simulink model "Type2_b"  (R2019a)
settings: Solver=VariableStepAuto  StartTime=0.0  StopTime=10.0  RelTol=1e-3
libraries: simulink x2
settings Model: Creator=admin  LastModifiedBy=admin

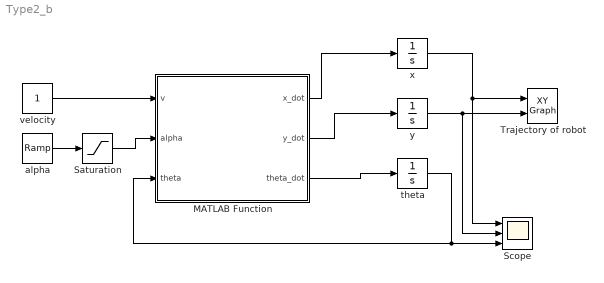
== system Type2_b ==
  MATLAB Function : MATLAB Function  TreatAsAtomicUnit=on
  Saturation : Saturate  UpperLimit=pi/4  LowerLimit=-pi/4
  Scope : Scope  NumInputPorts=3
  Trajectory of robot : simulink/Sinks/XY Graph  xmin=-1  xmax=5  ymin=-1  ymax=7  st=-1
  alpha : simulink/Sources/Ramp  slope=0.5  start=0  InitialOutput=0
  theta : Integrator
  velocity : Constant
  x : Integrator
  y : Integrator
  wires:
  MATLAB Function/1(x_dot) -> x/1
  theta/1 -> Scope/3, MATLAB Function/3(theta)
  MATLAB Function/2(y_dot) -> y/1
  x/1 -> Scope/1, Trajectory of robot/1
  y/1 -> Scope/2, Trajectory of robot/2
  MATLAB Function/3(theta_dot) -> theta/1
  velocity/1 -> MATLAB Function/1(v)
  alpha/1 -> Saturation/1
  Saturation/1 -> MATLAB Function/2(alpha)

== matlab function Type2_b/MATLAB Function ==
  data: v input; x_dot output; alpha input; theta input; y_dot output; theta_dot output
function [x_dot, y_dot, theta_dot] = tricycle_type_2(v, alpha, theta)
d = sqrt(3.1);
x_dot = v*cos(theta);
y_dot = v*sin(theta);
theta_dot = v/d*tan(alpha);
